simulink model "test_inverters"  (R2025b)
settings: Solver=VariableStepAuto  StartTime=0.0  StopTime=5/60  RelTol=1e-3
libraries: fl_lib x13, ee_lib_for_power_systems x12, nesl_utility x6, ee_lib x6, eePwmGeneratorTwoLevel x4, eeGeneralControl x1
settings Model: Creator=gdudgeon  LastModifiedBy=gdudgeon
settings RTWCC: GPUComputeCapability=3.5

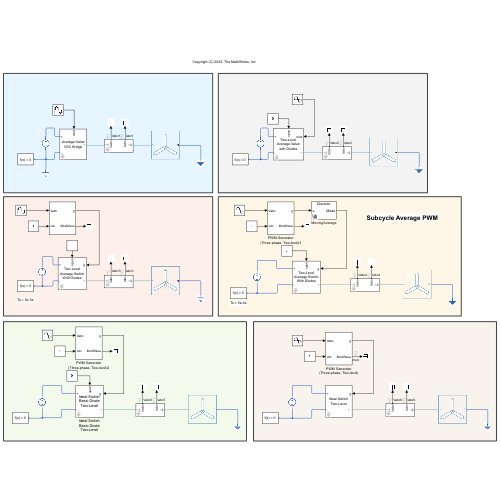
[thumbnail: Simulink's stored preview of the top-level diagram]
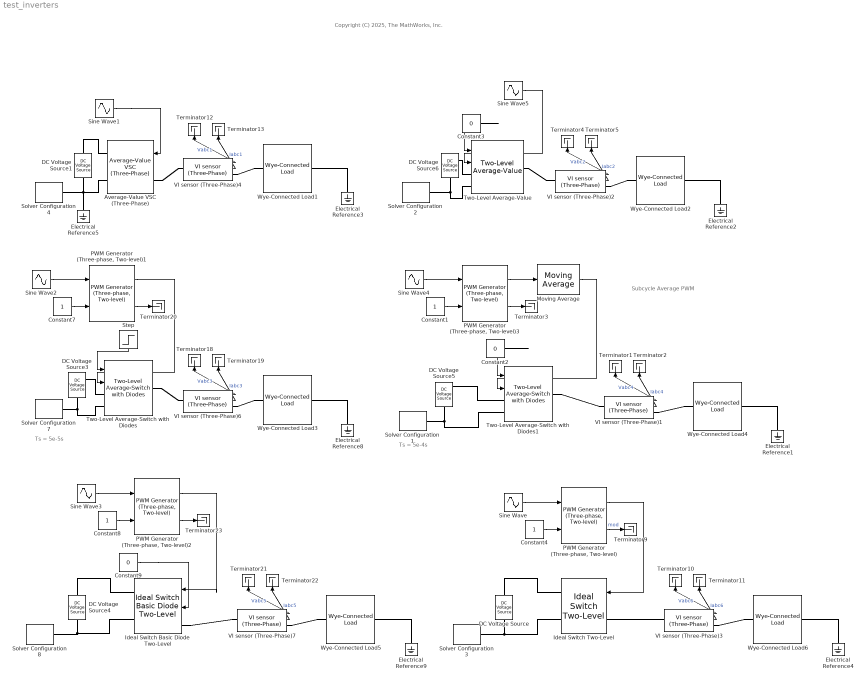
== system test_inverters ==
  note: Ts = 5e-4s
  note: Copyright (C) 2025, The MathWorks, Inc.
  note: Subcycle Average PWM
  note: Ts = 5e-5s
  Average-Value VSC (Three-Phase) : ee_lib_for_power_systems/Power Converters/Average-Value VSC (Three-Phase)  Ploss=1  run_time=off
      settings: SourceProductName=Support Library for Power Systems
  Constant{1,4,7..8} (4 alike) : Constant  SampleTime=-1
  Constant2 : Constant  Value=0  SampleTime=-1
  Constant3 : Constant  Value=0  SampleTime=-1
  Constant9 : Constant  Value=0  SampleTime=-1
  DC Voltage Source{,1,3..6} (6 alike) : fl_lib/Electrical/Electrical Sources/DC Voltage Source  v0=100 V
  Electrical Reference{1..5,8..9} (7 alike) : fl_lib/Electrical/Electrical Elements/Electrical Reference
  Ideal Switch Basic Diode Two-Level : ee_lib_for_power_systems/Power Converters/Ideal Switch Basic Diode Two-Level  Ron=1e-3  Goff=1e-6
      settings: SourceProductName=Support Library for Power Systems
  Ideal Switch Two-Level : ee_lib_for_power_systems/Power Converters/Ideal Switch Two-Level  Vf=1e-3  Ron=1e-3  Goff=1e-6  run_time=off
      settings: SourceProductName=Support Library for Power Systems
  Moving Average : eeGeneralControl/Moving Average  VariantControl=Variant1  LabelModeActiveChoice=Discrete  f=1/5e-4  x0=0  BufferSize=8192  Ts=50e-6
      settings: LibrarySourceBlock=ee_sl_lib/General Control/Moving Average
  PWM Generator (Three-phase, Two-level){,1..3} (4 alike) : eePwmGeneratorTwoLevel/PWM Generator (Three-phase, Two-level)  PWMMode=Continuous PWM (CPWM)  CPWMMode=SPWM: sinusoidal PWM  DPWMMode=60 DPWM: 60 degree discontinuous PWM  fsw=2e3  Ts=5e-5
      settings: LibrarySourceBlock=|
      | ee_sl_lib/Pulse Width
      | Modulation/PWM Generator
      | (Three-phase, Two-level)
  Sine Wave{,2..4} (4 alike) : Sin  Amplitude=0.5  Frequency=120*pi  Phase=[0 -1 1]*2*pi/3  SampleTime=50e-6
  Sine Wave1 : Sin  Frequency=120*pi  Phase=[0 -1 1]*2*pi/3  SampleTime=50e-6
  Sine Wave5 : Sin  Frequency=120*pi  Phase=[0 -1 1]*2*pi/3  SampleTime=50e-6
  Solver Configuration 1 : nesl_utility/Solver Configuration  PhysicalDomain=network_engine_domain  SubClassName=solver  LeftPortType=input  RightPortType=generic  Tones=[]  Harmonics=[]  SimulateNoise=off  Profile=off  UseLocalSampling=off  EnableSwitchedLinearOptims=on  FrequencyDomain=off  UseCCode=off  RelTol=0.001  AbsTol=0.001  MinStep=1e-09  ToWorkspace=off  RevertToSquareIcSolve=off  NumHomotopyIterations=100  PhasorMode=off  PhasorModeNumHarmonics=1  ConsistencySolver=NEWTON_XTOL_AFTER_FTOL  IndexReductionMethod=None  DoDC=off  ResidualTolerance=1e-09  ConsistencyTolSource=GLOBAL  ConsistencyAbsTol=0.001  ConsistencyRelTol=0.001  ConsistencyTolFactor=0.001  UseLocalSolver=on  LocalSolverChoice=NE_PARTITIONING_ADVANCER  ResolveIndetEquations=off  FunctionEvalNumThread=1  LocalSolverSampleTime=1e-4  DoFixedCost=off  MaxNonlinIter=2  MaxModeIter=2  ComputeImpulses=off  ImpulseIterations=2  LinearAlgebra=Sparse  LinearAlgebraNumThread=0  EquationFormulation=NE_TIME_EF  DelaysMemoryBudget=1024  AutomaticFiltering=off  FilteringTimeConstant=0.001  PartitionStorageMethod=AS_NEEDED  PartitionMemoryBudget=1024  PartitionMethod=ROBUST  MultibodyUseLocalSolver=off  MultibodyLocalSolverChoice=ODE1  MultibodyLocalSolverSampleTime=0.001
  Solver Configuration {2..4,7..8} (5 alike) : nesl_utility/Solver Configuration  PhysicalDomain=network_engine_domain  SubClassName=solver  LeftPortType=input  RightPortType=generic  Tones=[]  Harmonics=[]  SimulateNoise=off  Profile=off  UseLocalSampling=off  EnableSwitchedLinearOptims=on  FrequencyDomain=off  UseCCode=off  RelTol=0.001  AbsTol=0.001  MinStep=1e-09  ToWorkspace=off  RevertToSquareIcSolve=off  NumHomotopyIterations=100  PhasorMode=off  PhasorModeNumHarmonics=1  ConsistencySolver=NEWTON_XTOL_AFTER_FTOL  IndexReductionMethod=None  DoDC=off  ResidualTolerance=1e-09  ConsistencyTolSource=GLOBAL  ConsistencyAbsTol=0.001  ConsistencyRelTol=0.001  ConsistencyTolFactor=0.001  UseLocalSolver=on  LocalSolverChoice=NE_PARTITIONING_ADVANCER  ResolveIndetEquations=off  FunctionEvalNumThread=1  LocalSolverSampleTime=50e-6  DoFixedCost=off  MaxNonlinIter=2  MaxModeIter=2  ComputeImpulses=off  ImpulseIterations=2  LinearAlgebra=Sparse  LinearAlgebraNumThread=0  EquationFormulation=NE_TIME_EF  DelaysMemoryBudget=1024  AutomaticFiltering=off  FilteringTimeConstant=0.001  PartitionStorageMethod=AS_NEEDED  PartitionMemoryBudget=1024  PartitionMethod=ROBUST  MultibodyUseLocalSolver=off  MultibodyLocalSolverChoice=ODE1  MultibodyLocalSolverSampleTime=0.001
  Step : Step  Time=2.5/60  SampleTime=0
  Terminator{1..5,9..13,18..23} (16 alike) : Terminator
  Two-Level Average-Switch with Diodes : ee_lib_for_power_systems/Power Converters/Two-Level Average-Switch with Diodes  Vf=1e-3  Ron=1e-3  Goff=1e-6
      settings: SourceProductName=Support Library for Power Systems
  Two-Level Average-Switch with Diodes1 : ee_lib_for_power_systems/Power Converters/Two-Level Average-Switch with Diodes  Vf=1e-3  Ron=1e-5  Goff=1e-5
      settings: SourceProductName=Support Library for Power Systems
  Two-Level Average-Value : ee_lib_for_power_systems/Power Converters/Two-Level Average-Value  Vf=1e-3  Ron=1e-5  Goff=1e-5
      settings: SourceProductName=Support Library for Power Systems
  VI sensor (Three-Phase){1..4,6..7} (6 alike) : ee_lib_for_power_systems/Sense and Measure/VI sensor (Three-Phase)  volt_meas=Line-to-Line (Line Voltage)  meas_units=SI  Vnom=24e3  Pnom=100e6
      settings: SourceProductName=Support Library for Power Systems
  Wye-Connected Load{1..6} (6 alike) : ee_lib/Passive/RLC Assemblies/Wye-Connected Load  port_option=ee.enum.threePhasePort.composite  parameterization=ee.enum.rlc.parameterization.ratedpower  component_structure=ee.enum.rlc.structure.R  component_structure_PQ=ee.enum.rlc.structure.SeriesRL  R=1 Ohm  L=1e-3 H  C=1e-6 F  VRated=100*sqrt(3/2) V  FRated=60 Hz  P=1e5 W  Qpos=1e4 A*V  Qneg=-1e2 A*V  R_parasitic=0 Ohm  G_parasitic=0 1/Ohm  R_parasitic_PQ=0 Ohm  G_parasitic_PQ=0 1/Ohm  Vmag0=24e3 V  Vang0=0 deg  Freq0=60 Hz  IL_specify=off  IL_priority=High  IL=[0, 0, 0] A  IL_nominal_specify=off  IL_nominal_value=1  IL_nominal_unit=A  VC_specify=off  VC_priority=High  VC=[0, 0, 0] V  VC_nominal_specify=off  VC_nominal_value=1  VC_nominal_unit=V
  wires:
  "PWM Generator (Three-phase, Two-level)"/1 -> Ideal Switch Two-Level/1
  "PWM Generator (Three-phase, Two-level)"/2 -> Terminator9/1  "mod"
  Constant4/1 -> "PWM Generator (Three-phase, Two-level)"/2
  Sine Wave/1 -> "PWM Generator (Three-phase, Two-level)"/1
  VI sensor (Three-Phase)3/1 -> Terminator10/1  "Vabc6"
  VI sensor (Three-Phase)3/2 -> Terminator11/1  "Iabc6"
  VI sensor (Three-Phase)4/2 -> Terminator13/1  "Iabc1"
  VI sensor (Three-Phase)4/1 -> Terminator12/1  "Vabc1"
  Sine Wave1/1 -> Average-Value VSC (Three-Phase)/1
  VI sensor (Three-Phase)6/1 -> Terminator18/1  "Vabc3"
  VI sensor (Three-Phase)6/2 -> Terminator19/1  "Iabc3"
  Step/1 -> Two-Level Average-Switch with Diodes/1
  Sine Wave2/1 -> "PWM Generator (Three-phase, Two-level)1"/1
  Constant7/1 -> "PWM Generator (Three-phase, Two-level)1"/2
  "PWM Generator (Three-phase, Two-level)1"/2 -> Terminator20/1
  "PWM Generator (Three-phase, Two-level)1"/1 -> Two-Level Average-Switch with Diodes/2
  VI sensor (Three-Phase)7/2 -> Terminator22/1  "Iabc5"
  VI sensor (Three-Phase)7/1 -> Terminator21/1  "Vabc5"
  Sine Wave3/1 -> "PWM Generator (Three-phase, Two-level)2"/1
  Constant8/1 -> "PWM Generator (Three-phase, Two-level)2"/2
  "PWM Generator (Three-phase, Two-level)2"/2 -> Terminator23/1
  "PWM Generator (Three-phase, Two-level)2"/1 -> Ideal Switch Basic Diode Two-Level/1
  Constant9/1 -> Ideal Switch Basic Diode Two-Level/2
  Constant2/1 -> Two-Level Average-Switch with Diodes1/1
  "PWM Generator (Three-phase, Two-level)3"/2 -> Terminator3/1
  Constant1/1 -> "PWM Generator (Three-phase, Two-level)3"/2
  Sine Wave4/1 -> "PWM Generator (Three-phase, Two-level)3"/1
  VI sensor (Three-Phase)1/1 -> Terminator1/1  "Vabc4"
  VI sensor (Three-Phase)1/2 -> Terminator2/1  "Iabc4"
  "PWM Generator (Three-phase, Two-level)3"/1 -> Moving Average/1
  Moving Average/1 -> Two-Level Average-Switch with Diodes1/2
  VI sensor (Three-Phase)2/1 -> Terminator4/1  "Vabc2"
  VI sensor (Three-Phase)2/2 -> Terminator5/1  "Iabc2"
  Sine Wave5/1 -> Two-Level Average-Value/2
  Constant3/1 -> Two-Level Average-Value/1
  connections:
  DC Voltage Source/LConn1 -- Ideal Switch Two-Level/RConn1
  DC Voltage Source/RConn1 -- Solver Configuration 3/RConn1 -- Ideal Switch Two-Level/RConn2
  VI sensor (Three-Phase)3/LConn1 -- Ideal Switch Two-Level/LConn1
  Wye-Connected Load6/LConn1 -- VI sensor (Three-Phase)3/RConn1
  Wye-Connected Load6/RConn1 -- Electrical Reference4/LConn1
  DC Voltage Source1/RConn1 -- Solver Configuration 4/RConn1 -- Electrical Reference5/LConn1 -- Average-Value VSC (Three-Phase)/RConn2
  Electrical Reference3/LConn1 -- Wye-Connected Load1/RConn1
  Wye-Connected Load1/LConn1 -- VI sensor (Three-Phase)4/RConn1
  Average-Value VSC (Three-Phase)/LConn1 -- VI sensor (Three-Phase)4/LConn1
  Average-Value VSC (Three-Phase)/RConn1 -- DC Voltage Source1/LConn1
  DC Voltage Source3/RConn1 -- Solver Configuration 7/RConn1 -- Two-Level Average-Switch with Diodes/LConn2
  Two-Level Average-Switch with Diodes/LConn1 -- DC Voltage Source3/LConn1
  Two-Level Average-Switch with Diodes/RConn1 -- VI sensor (Three-Phase)6/LConn1
  Wye-Connected Load3/LConn1 -- VI sensor (Three-Phase)6/RConn1
  Wye-Connected Load3/RConn1 -- Electrical Reference8/LConn1
  DC Voltage Source4/RConn1 -- Solver Configuration 8/RConn1 -- Ideal Switch Basic Diode Two-Level/RConn2
  Wye-Connected Load5/LConn1 -- VI sensor (Three-Phase)7/RConn1
  Ideal Switch Basic Diode Two-Level/LConn1 -- VI sensor (Three-Phase)7/LConn1
  Wye-Connected Load5/RConn1 -- Electrical Reference9/LConn1
  Ideal Switch Basic Diode Two-Level/RConn1 -- DC Voltage Source4/LConn1
  DC Voltage Source5/RConn1 -- Two-Level Average-Switch with Diodes1/LConn2 -- Solver Configuration 1/RConn1
  Two-Level Average-Switch with Diodes1/LConn1 -- DC Voltage Source5/LConn1
  Wye-Connected Load4/RConn1 -- Electrical Reference1/LConn1
  Two-Level Average-Switch with Diodes1/RConn1 -- VI sensor (Three-Phase)1/LConn1
  Wye-Connected Load4/LConn1 -- VI sensor (Three-Phase)1/RConn1
  DC Voltage Source6/RConn1 -- Solver Configuration 2/RConn1 -- Two-Level Average-Value/LConn2
  VI sensor (Three-Phase)2/LConn1 -- Two-Level Average-Value/RConn1
  Wye-Connected Load2/LConn1 -- VI sensor (Three-Phase)2/RConn1
  Wye-Connected Load2/RConn1 -- Electrical Reference2/LConn1
  Two-Level Average-Value/LConn1 -- DC Voltage Source6/LConn1
